simulink model "sim04"  (R2012b)
settings: Solver=ode45  StartTime=0.0  StopTime=10.0  RelTol=1e-3
settings Model: Creator=Administrator  LastModifiedBy=Administrator

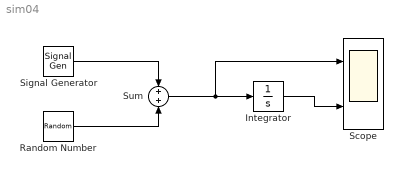
== system sim04 ==
  Integrator : Integrator
  Random Number : RandomNumber  Variance=0.2  SampleTime=0.1
  Scope : Scope  NumInputPorts=2
      settings: YMin=-5~-5  YMax=5~5
  Signal Generator : SignalGenerator  WaveForm=sawtooth  Amplitude=4  Frequency=3  Units=rad/sec
  Sum : Sum
  wires:
  Signal Generator/1 -> Sum/1
  Random Number/1 -> Sum/2
  Sum/1 -> Scope/1, Integrator/1
  Integrator/1 -> Scope/2
